simulink model "edrive"  (R2016b)
settings: Solver=ode1  StartTime=0.0  StopTime=1  FixedStep=ctrlConst.TsSim  MaxStep=1e-6  RelTol=1e-3  EnableMultiTasking=on
PreLoadFcn:
  | %rtwdemo_pmsmfoc_data
StartFcn:
  | %clear executionProfile
StopFcn:
  | %try
  | %  AddExecutionProfileToDataInspector();
  | %end
undefined symbols (not defined in the file or in its folder): canChannel, ctrlConst, ECM, EGM, hm11, hm13, hm5, hm7, Np, pmsm, sensors, sldrtexcb_modeswitch, SpdSetTest, theta0, TrqSetTest, Ts_10ms, Tsw
libraries: powerlib x26, canmsglib x23, simulink x14, canlib x12, powerlib_extras x9
(part 2 of 4)

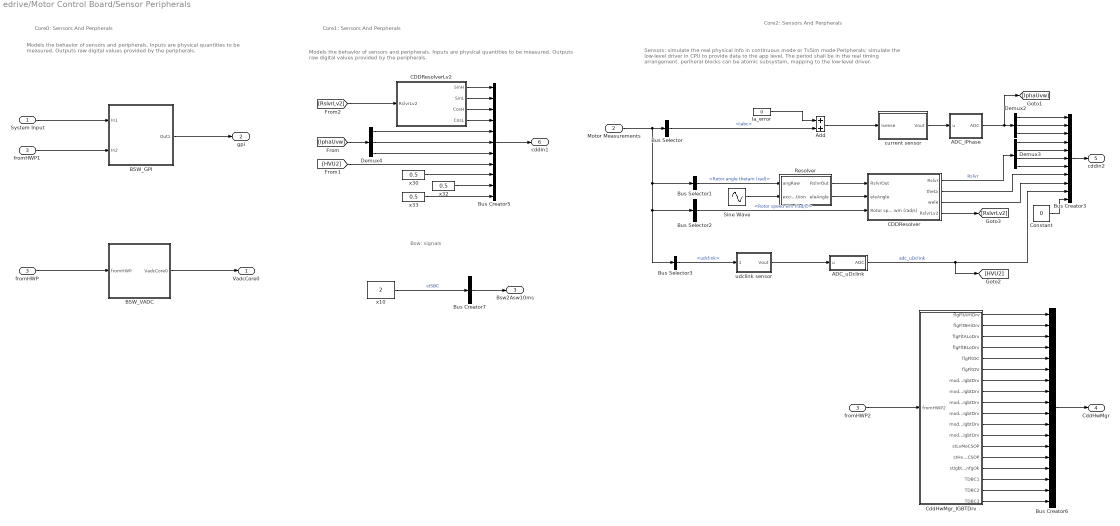
== system edrive/Motor Control Board/Sensor Peripherals ==
  note: Models the behavior of sensors and peripherals.
      | Inputs are physical quantities to be measured. Outputs raw digital values provided by the peripherals.
  note: Core0: Sensors And Perpherals
  note: Sensors: simulate the real physical info in continuous mode or TsSim mode
      | Peripherals: simulate the low-level driver in CPU to provide data to the app level. The period shall be in the real timing arrangement.
      | periheral blocks can be atomic subsystem, mapping to the low-level driver.
  note: Core2: Sensors And Perpherals
  note: Models the behavior of sensors and peripherals.
      | Inputs are physical quantities to be measured. Outputs raw digital values provided by the peripherals.
  note: Bsw: signals
  note: Core1: Sensors And Perpherals
  System Input : Inport
  Motor Measurements : Inport  Port=2
  fromHWP : Inport  Port=3
  ADC_iPhase : Subsystem
  ADC_uDclink : Subsystem
  Add : Sum
  BSW_GPI : Subsystem
  BSW_VADC : Subsystem
  Bus Creator3 : BusCreator  Inputs=11
  Bus Creator5 : BusCreator  Inputs=11
  Bus Creator6 : BusCreator  Inputs=18  OutDataTypeStr=Bus: CDDHwMgrST
  Bus Creator7 : BusCreator  Inputs=1
  Bus Selector : BusSelector  OutputSignals=electrical_measurements.Iabc
  Bus Selector1 : BusSelector  OutputSignals=mechanical_measurements.Rotor angle thetam (rad)
  Bus Selector2 : BusSelector  OutputSignals=mechanical_measurements.Rotor speed wm (rad/s)
  Bus Selector3 : BusSelector  OutputSignals=electrical_measurements.udclink
  CDDResolver : Subsystem
  CDDResolverLv2 : Subsystem
  CddHwMgr_IGBTDrv : Subsystem
  Constant : Constant  Value=0  OutDataTypeStr=uint16
  Demux2 : Demux  Outputs=3
  Demux3 : Demux
  Demux4 : Demux  Outputs=3
  Ia_error : Constant  Value=0
  Resolver : Subsystem
  Sine Wave : Sin  Amplitude=10  Frequency=10e3*2*pi  SampleTime=0
  current sensor : Subsystem
  fromHWP1 : InportShadow  Port=3
  fromHWP2 : InportShadow  Port=3
  udclink sensor : Subsystem
  x10 : Constant  Value=2  OutDataTypeStr=uint16
      settings: AttributesFormatString=DT: %<OutDataTypeStr>
  x30 : Constant  Value=0.5  OutDataTypeStr=single
      settings: AttributesFormatString=DT: %<OutDataTypeStr>
  x32 : Constant  Value=0.5  OutDataTypeStr=single
      settings: AttributesFormatString=DT: %<OutDataTypeStr>
  x33 : Constant  Value=0.5  OutDataTypeStr=single
      settings: AttributesFormatString=DT: %<OutDataTypeStr>
  VadcCore0 : Outport  OutDataTypeStr=Bus: VADCST
  gpi : Outport  Port=2  OutDataTypeStr=Bus: GPIST
  Bsw2Asw10ms : Outport  Port=3  OutDataTypeStr=Bus: Bsw2Asw10msST
  CddHwMgr : Outport  Port=4
  cddin2 : Outport  Port=5  OutDataTypeStr=Bus: CDDIN2ST
  cddin1 : Outport  Port=6  OutDataTypeStr=Bus: CDDIN1ST
  wires:
  Bus Creator6/1 -> CddHwMgr/1
  Bus Selector1/1 -> Resolver/1(angRaw)  "<Rotor angle thetam (rad)>"
  Sine Wave/1 -> Resolver/2(excitatiion)
  Motor Measurements/1 -> Bus Selector3/1, Bus Selector2/1, Bus Selector1/1, Bus Selector/1
  current sensor/1(Vout) -> ADC_iPhase/1(u)
  udclink sensor/1(Vout) -> ADC_uDclink/1(u)
  Bus Selector3/1 -> udclink sensor/1(uSense)  "<udclink>"
  Resolver/1(RslvrOut) -> CDDResolver/1(RslvrOut)
  Resolver/2(eleAngle) -> CDDResolver/2(eleAngle)
  Bus Selector2/1 -> CDDResolver/3(Rotor speed wm (rad/s))  "<Rotor speed wm (rad/s)>"
  Bus Selector/1 -> Add/2  "<Iabc>"
  ADC_uDclink/1(ADC) -> Bus Creator3/10, [HVU2]  "adc_uDclink"
  CDDResolver/1(Rslvr) -> Demux3/1  "Rslvr"
  Ia_error/1 -> Add/1
  Bus Creator5/1 -> cddin1/1
  [HVU2] -> Bus Creator5/8
  ADC_iPhase/1(ADC) -> [IphaUvw], Demux2/1
  [IphaUvw] -> Demux4/1
  Demux4/1 -> Bus Creator5/5
  Demux4/2 -> Bus Creator5/6
  Demux4/3 -> Bus Creator5/7
  CDDResolver/4(RslvrLv2) -> [RslvrLv2]
  CDDResolverLv2/1(SinH) -> Bus Creator5/1
  CDDResolverLv2/2(SinL) -> Bus Creator5/2
  CDDResolverLv2/3(CosH) -> Bus Creator5/3
  CDDResolverLv2/4(CosL) -> Bus Creator5/4
  [RslvrLv2] -> CDDResolverLv2/1(RslvrLv2)
  Bus Creator7/1 -> Bsw2Asw10ms/1
  x10/1 -> Bus Creator7/1  "stSBC"
  Add/1 -> current sensor/1(Isense)
  x30/1 -> Bus Creator5/9
  x32/1 -> Bus Creator5/10
  x33/1 -> Bus Creator5/11
  CddHwMgr_IGBTDrv/1(flgFltAHiDrv) -> Bus Creator6/1
  CddHwMgr_IGBTDrv/3(flgFltALoDrv) -> Bus Creator6/3
  CddHwMgr_IGBTDrv/4(flgFltBLoDrv) -> Bus Creator6/4
  CddHwMgr_IGBTDrv/5(flgFltOC) -> Bus Creator6/5
  CddHwMgr_IGBTDrv/6(flgFltOV) -> Bus Creator6/6
  CddHwMgr_IGBTDrv/13(stLvMoCSOP) -> Bus Creator6/13
  CddHwMgr_IGBTDrv/2(flgFltBHiDrv) -> Bus Creator6/2
  CddHwMgr_IGBTDrv/9(modLo3IgbtDrv) -> Bus Creator6/9
  CddHwMgr_IGBTDrv/12(modHi3IgbtDrv) -> Bus Creator6/12
  CddHwMgr_IGBTDrv/11(modHi2IgbtDrv) -> Bus Creator6/11
  CddHwMgr_IGBTDrv/7(modLo1IgbtDrv) -> Bus Creator6/7
  CddHwMgr_IGBTDrv/8(modLo2IgbtDrv) -> Bus Creator6/8
  CddHwMgr_IGBTDrv/10(modHi1IgbtDrv) -> Bus Creator6/10
  CddHwMgr_IGBTDrv/14(stHvMoCSOP) -> Bus Creator6/14
  BSW_VADC/1(VadcCore0) -> VadcCore0/1
  fromHWP/1 -> BSW_VADC/1(fromHWP)
  fromHWP2/1 -> CddHwMgr_IGBTDrv/1(fromHWP2)
  CddHwMgr_IGBTDrv/15(stIgbtDrvCnfgOk) -> Bus Creator6/15
  Bus Creator3/1 -> cddin2/1
  Demux2/1 -> Bus Creator3/1
  Demux2/2 -> Bus Creator3/2
  Demux2/3 -> Bus Creator3/3
  Demux3/1 -> Bus Creator3/4
  Demux3/2 -> Bus Creator3/5
  Demux3/3 -> Bus Creator3/6
  Demux3/4 -> Bus Creator3/7
  CDDResolver/2(theta) -> Bus Creator3/8
  CDDResolver/3(wele) -> Bus Creator3/9
  Constant/1 -> Bus Creator3/11
  CddHwMgr_IGBTDrv/16(TDBC1) -> Bus Creator6/16
  CddHwMgr_IGBTDrv/17(TDBC2) -> Bus Creator6/17
  CddHwMgr_IGBTDrv/18(TDBC3) -> Bus Creator6/18
  System Input/1 -> BSW_GPI/1(In1)
  fromHWP1/1 -> BSW_GPI/2(In2)
  BSW_GPI/1(Out1) -> gpi/1

== system edrive/Power Inverter and Motor/Inverter ==
  note: Change UVW to Motor here
  note: Construct electrical waveforms for the three motor phases.
  note: Inverter
  gate1 : Inport
  Bus Creator : BusCreator  Inputs=3
  Current Measurement : powerlib/Measurements/Current Measurement  Tag=PoWeRsYsTeMmEaSuReMeNt  PhasorSimulation=off  OutputType=Magnitude  PSBequivalent=0
  DC Voltage Source1 : powerlib/Electrical Sources/DC Voltage Source  Amplitude=pmsm.Udc  Measurements=None
  IGBT  B6 : powerlib/Power Electronics/Universal Bridge  Arms=3  SnubberResistance=1e6  SnubberCapacitance=1e-9  Device=IGBT / Diodes  Ron=1.1e-3  Lon=0  ForwardVoltages="[0.7  0.7]"  ForwardVoltage=0  GTOparameters=[ 10e-6 , 20e-6 ]  IGBTparameters=[0.1e-6 , 0.1e-6 ]  Measurements=None  Measurements_2=None  converterType=Rectifier
  Measure : Subsystem
  RC1 : powerlib/Elements/Series RLC Branch  LConnTagsString=__new0  RConnTagsString=__new0  BranchType=RC  Resistance=0.001  Inductance=7e-9  SetiL0=off  InitialCurrent=0  Capacitance=500e-6  Setx0=on  InitialVoltage=pmsm.Udc  Measurements=None
  RC2 : powerlib/Elements/Series RLC Branch  LConnTagsString=__new0  RConnTagsString=__new0  BranchType=RL  Resistance=(45+2)*1e-3  Inductance=2.5e-6  SetiL0=off  InitialCurrent=0  Capacitance=500e-6  Setx0=off  InitialVoltage=0  Measurements=None
  Rshort : powerlib/Elements/Series RLC Branch  LConnTagsString=__new0  RConnTagsString=__new0  BranchType=R  Resistance=1e-5  Inductance=7e-9  SetiL0=off  InitialCurrent=0  Capacitance=500e-6  Setx0=on  InitialVoltage=330  Measurements=None
  A : PMIOPort  Port=1  Side=Right
  B : PMIOPort  Port=2  Side=Right
  C : PMIOPort  Port=3  Side=Right
  "EleMeasurement " : Outport
  wires:
  Current Measurement/1 -> Measure/1(Idc)
  Measure/2(I_abc) -> Bus Creator/2  "Iabc"
  Measure/3(Vdc) -> Bus Creator/3  "udclink"
  gate1/1 -> IGBT  B6/1
  Bus Creator/1 -> "EleMeasurement "/1
  Measure/1(Pdclnk) -> Bus Creator/1  "Pdclink"
  connections:
  DC Voltage Source1/LConn1 -- IGBT  B6/RConn2 -- Measure/LConn4 -- RC1/RConn1
  RC2/LConn1 -- RC1/LConn1 -- Measure/LConn5 -- Current Measurement/LConn1 -- Rshort/LConn1
  DC Voltage Source1/RConn1 -- RC2/RConn1 -- Rshort/RConn1
  A/RConn1 -- Measure/RConn1
  IGBT  B6/RConn1 -- Current Measurement/RConn1
  Measure/RConn2 -- B/RConn1
  Measure/RConn3 -- C/RConn1
  IGBT  B6/LConn2 -- Measure/LConn2
  IGBT  B6/LConn1 -- Measure/LConn1
  IGBT  B6/LConn3 -- Measure/LConn3

== system edrive/Power Inverter and Motor/Motor_feishi150 ==
  note: Motor
  note: Models the PMSM and outputs physical quantities used by the controller and visualizations.
      | The rotor position angle returned by the SimPowerSystems model must be offset to align with the reference angle that the controller expects.
      | Signal conversion blocks are used to enable renaming signals measured from the motor model.
  MotorMode : Inport
  Speed or Torque : Inport  Port=2
  Gain12 : Gain  Gain=2*pi/60
  PMSM : Subsystem
  A : PMIOPort  Port=1  Side=Left
  B : PMIOPort  Port=2  Side=Left
  C : PMIOPort  Port=3  Side=Left
  MotorMeasure : Outport
  wires:
  Speed or Torque/1 -> Gain12/1
  PMSM/1(m) -> MotorMeasure/1
  Gain12/1 -> PMSM/1(In)
  MotorMode/1 -> PMSM/2(MotorMode)
  connections:
  PMSM/LConn3 -- C/RConn1
  PMSM/LConn2 -- B/RConn1
  PMSM/LConn1 -- A/RConn1

== system edrive/System Analysis/Measure ==
  motor : Inport
  Bus Selector1 : BusSelector  OutputSignals=mechanical_measurements.Stator current is_q (A),mechanical_measurements.Stator current is_d (A),mechanical_measurements.Stator voltage Vs_q (V),mechanical_measurements.Stator voltage Vs_d (V),mechanical_measurements.Rotor speed wm (rad/s),mechanical_measurements.Electromagnetic torque Te (N*m),electrical_measurements.Pdclink
  Eff Cal : MATLAB Function  TreatAsAtomicUnit=on
  Gain : Gain  Gain=1/sqrt(2)
  Gain1 : Gain  Gain=1/sqrt(2)
  Loss : Scope  NumInputPorts=2
  Mux2 : Mux  Inputs=2
  Saturation : Saturate  UpperLimit=1  LowerLimit=0
  Subsystem : Subsystem
  Subsystem1 : Subsystem
  Subsystem3 : Subsystem
  Subsystem4 : Subsystem
  Transfer Fcn1 : TransferFcn  Numerator=[1/sqrt(2)]  Denominator=[0.001 1]
  Transfer Fcn2 : TransferFcn  Denominator=[0.01 1]
  Transfer Fcn3 : TransferFcn  Numerator=[1/sqrt(2)]  Denominator=[0.001 1]
  Torque : Outport
  speed : Outport  Port=2
  Current : Outport  Port=3
  Voltage : Outport  Port=4
  Power : Outport  Port=5
  effEDrive : Outport  Port=6
  wires:
  motor/1 -> Bus Selector1/1
  Bus Selector1/2 -> Gain1/1  "<Stator current is_d (A)>"
  Bus Selector1/1 -> Gain/1  "<Stator current is_q (A)>"
  Bus Selector1/4 -> Transfer Fcn1/1  "<Stator voltage Vs_d (V)>"
  Bus Selector1/3 -> Transfer Fcn3/1  "<Stator voltage Vs_q (V)>"
  Subsystem/1(Cur.) -> Current/1
  Subsystem1/1(Vol.) -> Voltage/1
  Transfer Fcn3/1 -> Subsystem3/2(vq), Subsystem1/1(vq)
  Transfer Fcn1/1 -> Subsystem1/2(vd), Subsystem3/1(vd)
  Bus Selector1/5 -> Subsystem4/1(In1)  "<Rotor speed wm (rad/s)>"
  Bus Selector1/6 -> Subsystem4/2(In2)  "<Electromagnetic torque Te (N*m)>"
  Subsystem4/1(Torque) -> Torque/1
  Subsystem4/2(speed) -> speed/1
  Gain/1 -> Subsystem3/4(iq), Subsystem/1(iq)
  Gain1/1 -> Subsystem/2(id), Subsystem3/3(id)
  Mux2/1 -> Power/1
  Subsystem4/3(M_Power) -> Eff Cal/1(m_power), Mux2/1
  Saturation/1 -> Loss/1, effEDrive/1
  Eff Cal/1(eff) -> Saturation/1
  Bus Selector1/7 -> Transfer Fcn2/1  "<Pdclink>"
  Transfer Fcn2/1 -> Loss/2, Mux2/2, Eff Cal/2(e_power)

== system edrive/System Analysis/System test ==
  torque_in : Inport
  Abs : Abs
  Data Type Conversion2 : DataTypeConversion  OutDataTypeStr=double
  Demux : Demux  Outputs=2
  Rate Transition1 : RateTransition  OutPortSampleTime=0.001
  Rate Transition2 : RateTransition  OutPortSampleTime=1e-2
  Rate Transition4 : RateTransition  OutPortSampleTime=1e-2
  Subtract : Sum  Inputs=-+
  To TrqErrRms : ToWorkspace  VariableName=TrqErrRms  SaveFormat=Timeseries  SampleTime=0.001
      settings: MaxDataPoints=50
  test : MATLAB Function  TreatAsAtomicUnit=on  SystemSampleTime=1e-2
  Out : Outport
  wires:
  test/1(out) -> Out/1
  Demux/2 -> Data Type Conversion2/1, Rate Transition4/1
  torque_in/1 -> Demux/1
  Subtract/1 -> Abs/1
  Abs/1 -> Rate Transition1/1
  Rate Transition4/1 -> test/2(torque_act)
  Data Type Conversion2/1 -> Subtract/2
  Demux/1 -> Rate Transition2/1, Subtract/1
  Rate Transition1/1 -> To TrqErrRms/1
  Rate Transition2/1 -> test/1(torqueSet)

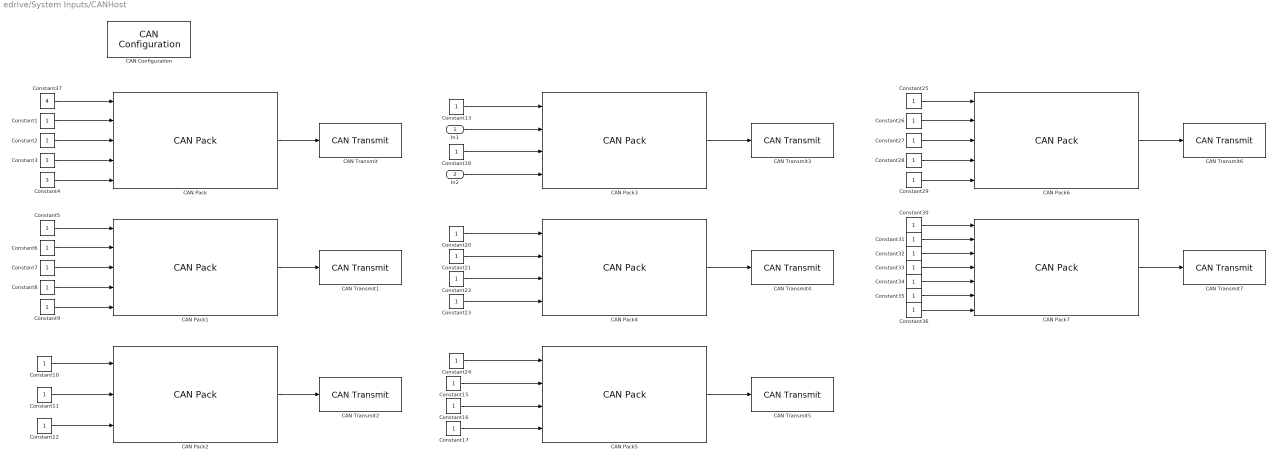
== system edrive/System Inputs/CANHost ==
  In1 : Inport
  In2 : Inport  Port=2
  CAN Configuration : canlib/CAN Configuration  BlockHandle=9440.0004  DeviceMenu=Kvaser Virtual 1 (Channel 2)  Device=Kvaser Virtual 1 (Channel 2)  ObjConstructor=canChannel('Kvaser', 'Virtual 1', 2)  BusSpeed=500000  EnableBitParameters=off  SJW=1  TSEG1=4  TSEG2=3  NSamples=1  AckMode=Normal
  CAN Pack : canmsglib/CAN Pack  CANdbFile=C:\MatlabWS\motorcontrol\controller\CAN_COM.dbc  MsgList=MSG_01  MsgName=MSG_01  MsgIDType=Standard (11-bit identifier)  MsgIdentifier=768  MsgLength=8  SignalInfo=MSG01_IdcMax$0$11$1$2$1$0$1$-1023$-1023$1024$#MSG01_IdcMin$11$11$1$2$1$0$1$-1023$-1023$1024$#MSG01_UdcMax$22$10$1$2$1$0$1$0$0$1023$#MSG01_UdcMin$32$10$1$2$1$0$1$0$0$1023$#MSG01_stHvbMaiRly$42$3$1$2$1$0$1$0$0$7$#  NSignals=5  StartBits=str2num('[int32(0);int32(11);int32(22);int32(32);int32(42)]')  SignalSizes=str2num('[int32(11);int32(11);int32(10);int32(10);int32(3)]')  ByteOrders=str2num('[int32(1);int32(1);int32(1);int32(1);int32(1)]')  DataTypes=str2num('[int32(2);int32(2);int32(2);int32(2);int32(2)]')  MultiplexTypes=str2num('[int32(1);int32(1);int32(1);int32(1);int32(1)]')  MultiplexValues=str2num('[double(0);double(0);double(0);double(0);double(0)]')  Factors=str2num('[double(1);double(1);double(1);double(1);double(1)]')  Offsets=str2num('[double(-1023);double(-1023);double(0);double(0);double(0)]')  Minimums=str2num('[double(-1023);double(-1023);double(0);double(0);double(0)]')  Maximums=str2num('[double(1024);double(1024);double(1023);double(1023);double(7)]')  Remote=off
      settings: DataFormat=CANdb specified signals
  CAN Pack1 : canmsglib/CAN Pack  CANdbFile=C:\MatlabWS\motorcontrol\controller\CAN_COM.dbc  MsgList=MSG_02  MsgName=MSG_02  MsgIDType=Standard (11-bit identifier)  MsgIdentifier=784  MsgLength=8  SignalInfo=MSG02_KpHigh$0$9$1$2$1$0$3.125000e-02$0$0$10$#MSG02_KpLow$9$9$1$2$1$0$3.125000e-02$0$0$10$#MSG02_NDeltaBound$18$16$1$2$1$0$5.000000e-01$-1.638350e+04$-1.638350e+04$16384$#MSG02_TrqPAmax$45$11$1$2$1$0$1$-1023$-1023$1024$#MSG02_TrqPAmin$34$11$1$2$1$0$1$-1023$-1023$1024$#  NSignals=5  StartBits=str2num('[int32(0);int32(9);int32(18);int32(45);int32(34)]')  SignalSizes=str2num('[int32(9);int32(9);int32(16);int32(11);int32(11)]')  ByteOrders=str2num('[int32(1);int32(1);int32(1);int32(1);int32(1)]')  DataTypes=str2num('[int32(2);int32(2);int32(2);int32(2);int32(2)]')  MultiplexTypes=str2num('[int32(1);int32(1);int32(1);int32(1);int32(1)]')  MultiplexValues=str2num('[double(0);double(0);double(0);double(0);double(0)]')  Factors=str2num('[double(3.125000e-02);double(3.125000e-02);double(5.000000e-01);double(1);double(1)]')  Offsets=str2num('[double(0);double(0);double(-1.638350e+04);double(-1023);double(-1023)]')  Minimums=str2num('[double(0);double(0);double(-1.638350e+04);double(-1023);double(-1023)]')  Maximums=str2num('[double(10);double(10);double(16384);double(1024);double(1024)]')  Remote=off
      settings: DataFormat=CANdb specified signals
  CAN Pack2 : canmsglib/CAN Pack  CANdbFile=C:\MatlabWS\motorcontrol\controller\CAN_COM.dbc  MsgList=MSG_03  MsgName=MSG_03  MsgIDType=Standard (11-bit identifier)  MsgIdentifier=800  MsgLength=8  SignalInfo=MSG03_TrqMax$0$11$1$2$1$0$1$-1023$-1023$1024$#MSG03_TrqMin$11$11$1$2$1$0$1$-1023$-1023$1024$#MSG03_cTrqSlopeMax$24$15$1$2$1$0$32$0$0$1048544$#  NSignals=3  StartBits=str2num('[int32(0);int32(11);int32(24)]')  SignalSizes=str2num('[int32(11);int32(11);int32(15)]')  ByteOrders=str2num('[int32(1);int32(1);int32(1)]')  DataTypes=str2num('[int32(2);int32(2);int32(2)]')  MultiplexTypes=str2num('[int32(1);int32(1);int32(1)]')  MultiplexValues=str2num('[double(0);double(0);double(0)]')  Factors=str2num('[double(1);double(1);double(32)]')  Offsets=str2num('[double(-1023);double(-1023);double(0)]')  Minimums=str2num('[double(-1023);double(-1023);double(0)]')  Maximums=str2num('[double(1024);double(1024);double(1048544)]')  Remote=off
      settings: DataFormat=CANdb specified signals
  CAN Pack3 : canmsglib/CAN Pack  CANdbFile=C:\MatlabWS\motorcontrol\controller\CAN_COM.dbc  MsgList=MSG_04  MsgName=MSG_04  MsgIDType=Standard (11-bit identifier)  MsgIdentifier=256  MsgLength=8  SignalInfo=MSG04_NSetP$0$16$1$2$1$0$1$-32767$-32767$32768$#MSG04_TrqSetP$20$11$1$2$1$0$1$-1023$-1023$1024$#MSG04_UdcSetP$32$10$1$2$1$0$1$0$0$1023$#MSG04_stModeReq$16$4$1$2$1$0$1$0$0$15$#  NSignals=4  StartBits=str2num('[int32(0);int32(20);int32(32);int32(16)]')  SignalSizes=str2num('[int32(16);int32(11);int32(10);int32(4)]')  ByteOrders=str2num('[int32(1);int32(1);int32(1);int32(1)]')  DataTypes=str2num('[int32(2);int32(2);int32(2);int32(2)]')  MultiplexTypes=str2num('[int32(1);int32(1);int32(1);int32(1)]')  MultiplexValues=str2num('[double(0);double(0);double(0);double(0)]')  Factors=str2num('[double(1);double(1);double(1);double(1)]')  Offsets=str2num('[double(-32767);double(-1023);double(0);double(0)]')  Minimums=str2num('[double(-32767);double(-1023);double(0);double(0)]')  Maximums=str2num('[double(32768);double(1024);double(1023);double(15)]')  Remote=off
      settings: DataFormat=CANdb specified signals
  CAN Pack4 : canmsglib/CAN Pack  CANdbFile=C:\MatlabWS\motorcontrol\controller\CAN_COM.dbc  MsgList=EM_05  MsgName=EM_05  MsgIDType=Standard (11-bit identifier)  MsgIdentifier=576  MsgLength=8  SignalInfo=EM05_FailCode1$0$16$1$2$1$0$1$0$0$65535$#EM05_FailCode2$16$16$1$2$1$0$1$0$0$65535$#EM05_FailCode3$32$16$1$2$1$0$1$0$0$65535$#EM05_FailCode4$48$16$1$2$1$0$1$0$0$65535$#  NSignals=4  StartBits=str2num('[int32(0);int32(16);int32(32);int32(48)]')  SignalSizes=str2num('[int32(16);int32(16);int32(16);int32(16)]')  ByteOrders=str2num('[int32(1);int32(1);int32(1);int32(1)]')  DataTypes=str2num('[int32(2);int32(2);int32(2);int32(2)]')  MultiplexTypes=str2num('[int32(1);int32(1);int32(1);int32(1)]')  MultiplexValues=str2num('[double(0);double(0);double(0);double(0)]')  Factors=str2num('[double(1);double(1);double(1);double(1)]')  Offsets=str2num('[double(0);double(0);double(0);double(0)]')  Minimums=str2num('[double(0);double(0);double(0);double(0)]')  Maximums=str2num('[double(65535);double(65535);double(65535);double(65535)]')  Remote=off
      settings: DataFormat=CANdb specified signals
  CAN Pack5 : canmsglib/CAN Pack  CANdbFile=C:\MatlabWS\motorcontrol\controller\CAN_COM.dbc  MsgList=MSG_06  MsgName=MSG_06  MsgIDType=Standard (11-bit identifier)  MsgIdentifier=288  MsgLength=8  SignalInfo=MSG06_TrqDmpLim$12$10$1$2$1$0$1$0$0$1023$#MSG06_TrqDmpMax$2$10$1$2$1$0$1$0$0$1023$#MSG06_kDmp$24$15$1$2$1$0$3.125000e-02$0$0$8$#MSG06_stDstCReq$0$2$1$2$1$0$1$0$0$3$#  NSignals=4  StartBits=str2num('[int32(12);int32(2);int32(24);int32(0)]')  SignalSizes=str2num('[int32(10);int32(10);int32(15);int32(2)]')  ByteOrders=str2num('[int32(1);int32(1);int32(1);int32(1)]')  DataTypes=str2num('[int32(2);int32(2);int32(2);int32(2)]')  MultiplexTypes=str2num('[int32(1);int32(1);int32(1);int32(1)]')  MultiplexValues=str2num('[double(0);double(0);double(0);double(0)]')  Factors=str2num('[double(1);double(1);double(3.125000e-02);double(1)]')  Offsets=str2num('[double(0);double(0);double(0);double(0)]')  Minimums=str2num('[double(0);double(0);double(0);double(0)]')  Maximums=str2num('[double(1023);double(1023);double(8);double(3)]')  Remote=off
      settings: DataFormat=CANdb specified signals
  CAN Pack6 : canmsglib/CAN Pack  CANdbFile=C:\MatlabWS\motorcontrol\controller\CAN_COM.dbc  MsgList=MSG_01  MsgName=MSG_01  MsgIDType=Standard (11-bit identifier)  MsgIdentifier=768  MsgLength=8  SignalInfo=MSG01_IdcMax$0$11$1$2$1$0$1$-1023$-1023$1024$#MSG01_IdcMin$11$11$1$2$1$0$1$-1023$-1023$1024$#MSG01_UdcMax$22$10$1$2$1$0$1$0$0$1023$#MSG01_UdcMin$32$10$1$2$1$0$1$0$0$1023$#MSG01_stHvbMaiRly$42$3$1$2$1$0$1$0$0$7$#  NSignals=5  StartBits=str2num('[int32(0);int32(11);int32(22);int32(32);int32(42)]')  SignalSizes=str2num('[int32(11);int32(11);int32(10);int32(10);int32(3)]')  ByteOrders=str2num('[int32(1);int32(1);int32(1);int32(1);int32(1)]')  DataTypes=str2num('[int32(2);int32(2);int32(2);int32(2);int32(2)]')  MultiplexTypes=str2num('[int32(1);int32(1);int32(1);int32(1);int32(1)]')  MultiplexValues=str2num('[double(0);double(0);double(0);double(0);double(0)]')  Factors=str2num('[double(1);double(1);double(1);double(1);double(1)]')  Offsets=str2num('[double(-1023);double(-1023);double(0);double(0);double(0)]')  Minimums=str2num('[double(-1023);double(-1023);double(0);double(0);double(0)]')  Maximums=str2num('[double(1024);double(1024);double(1023);double(1023);double(7)]')  Remote=off
      settings: DataFormat=CANdb specified signals
  CAN Pack7 : canmsglib/CAN Pack  CANdbFile=C:\MatlabWS\motorcontrol\controller\CAN_COM.dbc  MsgList=MSG_08  MsgName=MSG_08  MsgIDType=Extended (29-bit identifier)  MsgIdentifier=320  MsgLength=7  SignalInfo=MSG08_Alpha_Voltage_Cmd$8$8$1$2$1$0$1$0$0$255$#MSG08_Beta_Voltage_Cmd$16$8$1$2$1$0$1$0$0$255$#MSG08_D_Current_Cmd$48$8$1$2$1$0$1$0$0$255$#MSG08_D_Voltage_Cmd$24$8$1$2$1$0$1$0$0$255$#MSG08_Q_Current_Cmd$40$8$1$2$1$0$1$0$0$255$#MSG08_Q_Volatge_Cmd$32$8$1$2$1$0$1$0$0$255$#MSG08_control_mode$0$3$1$2$1$0$1$0$0$7$#  NSignals=7  StartBits=str2num('[int32(8);int32(16);int32(48);int32(24);int32(40);int32(32);int32(0)]')  SignalSizes=str2num('[int32(8);int32(8);int32(8);int32(8);int32(8);int32(8);int32(3)]')  ByteOrders=str2num('[int32(1);int32(1);int32(1);int32(1);int32(1);int32(1);int32(1)]')  DataTypes=str2num('[int32(2);int32(2);int32(2);int32(2);int32(2);int32(2);int32(2)]')  MultiplexTypes=str2num('[int32(1);int32(1);int32(1);int32(1);int32(1);int32(1);int32(1)]')  MultiplexValues=str2num('[double(0);double(0);double(0);double(0);double(0);double(0);double(0)]')  Factors=str2num('[double(1);double(1);double(1);double(1);double(1);double(1);double(1)]')  Offsets=str2num('[double(0);double(0);double(0);double(0);double(0);double(0);double(0)]')  Minimums=str2num('[double(0);double(0);double(0);double(0);double(0);double(0);double(0)]')  Maximums=str2num('[double(255);double(255);double(255);double(255);double(255);double(255);double(7)]')  Remote=off
      settings: DataFormat=CANdb specified signals
  CAN Transmit : canlib/CAN Transmit  BlockHandle=9449.0004  DeviceMenu=Kvaser Virtual 1 (Channel 2)  Device=Kvaser Virtual 1 (Channel 2)  ObjConstructor=canChannel('Kvaser', 'Virtual 1', 2)  EnablePeriodicTransmit=on  MessagePeriod=0.01
  CAN Transmit1 : canlib/CAN Transmit  BlockHandle=9450.0004  DeviceMenu=Kvaser Virtual 1 (Channel 2)  Device=Kvaser Virtual 1 (Channel 2)  ObjConstructor=canChannel('Kvaser', 'Virtual 1', 2)  EnablePeriodicTransmit=on  MessagePeriod=0.01
  CAN Transmit2 : canlib/CAN Transmit  BlockHandle=9451.0004  DeviceMenu=Kvaser Virtual 1 (Channel 2)  Device=Kvaser Virtual 1 (Channel 2)  ObjConstructor=canChannel('Kvaser', 'Virtual 1', 2)  EnablePeriodicTransmit=on  MessagePeriod=0.01
  CAN Transmit3 : canlib/CAN Transmit  BlockHandle=9452.0004  DeviceMenu=Kvaser Virtual 1 (Channel 2)  Device=Kvaser Virtual 1 (Channel 2)  ObjConstructor=canChannel('Kvaser', 'Virtual 1', 2)  EnablePeriodicTransmit=on  MessagePeriod=0.01
  CAN Transmit4 : canlib/CAN Transmit  BlockHandle=9453.0004  DeviceMenu=Kvaser Virtual 1 (Channel 2)  Device=Kvaser Virtual 1 (Channel 2)  ObjConstructor=canChannel('Kvaser', 'Virtual 1', 2)  EnablePeriodicTransmit=on  MessagePeriod=0.01
  CAN Transmit5 : canlib/CAN Transmit  BlockHandle=9454.0004  DeviceMenu=Kvaser Virtual 1 (Channel 2)  Device=Kvaser Virtual 1 (Channel 2)  ObjConstructor=canChannel('Kvaser', 'Virtual 1', 2)  EnablePeriodicTransmit=on  MessagePeriod=0.01
  CAN Transmit6 : canlib/CAN Transmit  BlockHandle=9455.0004  DeviceMenu=Kvaser Virtual 1 (Channel 2)  Device=Kvaser Virtual 1 (Channel 2)  ObjConstructor=canChannel('Kvaser', 'Virtual 1', 2)  EnablePeriodicTransmit=on  MessagePeriod=0.01
  CAN Transmit7 : canlib/CAN Transmit  BlockHandle=9456.0004  DeviceMenu=Kvaser Virtual 1 (Channel 2)  Device=Kvaser Virtual 1 (Channel 2)  ObjConstructor=canChannel('Kvaser', 'Virtual 1', 2)  EnablePeriodicTransmit=on  MessagePeriod=0.01
  Constant{1..3,5..13,15..18,20..36} (33 alike) : Constant
  Constant37 : Constant  Value=4
  Constant4 : Constant  Value=3
  wires:
  CAN Pack/1 -> CAN Transmit/1
  CAN Pack1/1 -> CAN Transmit1/1
  CAN Pack2/1 -> CAN Transmit2/1
  CAN Pack3/1 -> CAN Transmit3/1
  CAN Pack4/1 -> CAN Transmit4/1
  CAN Pack5/1 -> CAN Transmit5/1
  CAN Pack6/1 -> CAN Transmit6/1
  CAN Pack7/1 -> CAN Transmit7/1
  Constant37/1 -> CAN Pack/1
  Constant1/1 -> CAN Pack/2
  Constant2/1 -> CAN Pack/3
  Constant3/1 -> CAN Pack/4
  Constant4/1 -> CAN Pack/5
  Constant7/1 -> CAN Pack1/3
  Constant8/1 -> CAN Pack1/4
  Constant6/1 -> CAN Pack1/2
  Constant9/1 -> CAN Pack1/5
  Constant5/1 -> CAN Pack1/1
  Constant11/1 -> CAN Pack2/2
  Constant10/1 -> CAN Pack2/1
  Constant12/1 -> CAN Pack2/3
  Constant13/1 -> CAN Pack3/1
  In1/1 -> CAN Pack3/2
  Constant18/1 -> CAN Pack3/3
  In2/1 -> CAN Pack3/4
  Constant21/1 -> CAN Pack4/2
  Constant22/1 -> CAN Pack4/3
  Constant23/1 -> CAN Pack4/4
  Constant20/1 -> CAN Pack4/1
  Constant17/1 -> CAN Pack5/4
  Constant16/1 -> CAN Pack5/3
  Constant24/1 -> CAN Pack5/1
  Constant15/1 -> CAN Pack5/2
  Constant28/1 -> CAN Pack6/4
  Constant26/1 -> CAN Pack6/2
  Constant27/1 -> CAN Pack6/3
  Constant29/1 -> CAN Pack6/5
  Constant25/1 -> CAN Pack6/1
  Constant31/1 -> CAN Pack7/2
  Constant30/1 -> CAN Pack7/1
  Constant32/1 -> CAN Pack7/3
  Constant33/1 -> CAN Pack7/4
  Constant34/1 -> CAN Pack7/5
  Constant35/1 -> CAN Pack7/6
  Constant36/1 -> CAN Pack7/7

== system edrive/Motor Control Board/ComCanRxdGen/Subsystem1 ==
  In1 : Inport
  Terminator : Terminator
  Out1 : Outport
  wires:
  In1/1 -> Terminator/1
  [TrqInCan] -> Out1/1

== system edrive/Motor Control Board/ComCanRxdGen/Subsystem2 ==
  In1 : Inport
  Terminator : Terminator
  Out1 : Outport
  wires:
  [ModeInCan] -> Out1/1
  In1/1 -> Terminator/1

== system edrive/Motor Control Board/ComCanRxdGen/Subsystem3 ==
  In1 : Inport
  Terminator : Terminator
  Out1 : Outport
  wires:
  In1/1 -> Terminator/1
  [SpdInCan] -> Out1/1

== system edrive/Motor Control Board/GTM/SVPWMtoDuty ==
  note: Hoang Le-Huy
      | Universite Laval
      | Quebec
  note: Pierre Giroux, Gilbert Sybille
      | Power System Laboratory, IREQ
      | Hydro-Quebec
  note: Space Vector Pulse Width Modulation (SV PWM)
  tSwitch : Inport
  Demux2 : Demux  Outputs=12
  Generate pulse pattern : Subsystem
      mask init:
      | %Switching pattern:
      | pat1=[0 1 1 1 1 1 0;0 0 1 1 1 0 0;0 0 0 1 0 0 0];
      | pat1(:,:,2)=[0 0 1 1 1 0 0;0 1 1 1 1 1 0;0 0 0 1 0 0 0];
      | pat1(:,:,3)=[0 0 0 1 0 0 0;0 1 1 1 1 1 0;0 0 1 1 1 0 0];
      | pat1(:,:,4)=[0 0 0 1 0 0 0;0 0 1 1 1 0 0;0 1 1 1 1 1 0];
      | pat1(:,:,5)=[0 0 1 1 1 0 0;0 0 0 1 0 0 0;0 1 1 1 1 1 0];
      | pat1(:,:,6)=[0 1 1 1 1 1 0;0 0 0 1 0 0 0;0 0 1 1 1 0 0];
  Generate pulse pattern1 : Subsystem
      mask init: same as edrive/Motor Control Board/GTM/SVPWMtoDuty/Generate pulse pattern
  Generate pulse pattern2 : Subsystem
      mask init: same as edrive/Motor Control Board/GTM/SVPWMtoDuty/Generate pulse pattern
  Generate pulse pattern3 : Subsystem
      mask init: same as edrive/Motor Control Board/GTM/SVPWMtoDuty/Generate pulse pattern
  Generate pulse pattern4 : Subsystem
      mask init: same as edrive/Motor Control Board/GTM/SVPWMtoDuty/Generate pulse pattern
  Generate pulse pattern5 : Subsystem
      mask init: same as edrive/Motor Control Board/GTM/SVPWMtoDuty/Generate pulse pattern
  INFO : Subsystem
      mask Display: disp('?')
  Mux : Mux  Inputs=6
  Pulses : Outport
  wires:
  Generate pulse pattern5/1(TuLo) -> Mux/6
  Generate pulse pattern4/1(TuLo) -> Mux/4
  Generate pulse pattern1/1(TuHi) -> Mux/3
  Generate pulse pattern/1(TuHi) -> Mux/1
  Demux2/12 -> Generate pulse pattern5/2(TuLo_On)
  Demux2/11 -> Generate pulse pattern5/1(TuLo_Off)
  Demux2/10 -> Generate pulse pattern4/2(TuLo_On)
  Demux2/9 -> Generate pulse pattern4/1(TuLo_Off)
  Demux2/8 -> Generate pulse pattern3/2(TuLo_On)
  Demux2/7 -> Generate pulse pattern3/1(TuLo_Off)
  Demux2/6 -> Generate pulse pattern2/2(TuHi_Off)
  Demux2/5 -> Generate pulse pattern2/1(TuHi_On)
  Demux2/4 -> Generate pulse pattern1/2(TuHi_Off)
  Demux2/3 -> Generate pulse pattern1/1(TuHi_On)
  Demux2/2 -> Generate pulse pattern/2(TuHi_Off)
  Demux2/1 -> Generate pulse pattern/1(TuHi_On)
  tSwitch/1 -> Demux2/1
  Mux/1 -> Pulses/1
  Generate pulse pattern3/1(TuLo) -> Mux/2
  Generate pulse pattern2/1(TuHi) -> Mux/5

== system edrive/Motor Control Board/Sensor Peripherals/ADC_iPhase ==
  u : Inport
  ADC Volts To Driver Units : Constant  Value=sensors.ADC.VoltsToDriverUnits
  Driver Noise : Subsystem
      mask init:
      | if evalin('base','sensors.ADC.NoiseEnable')
      |     enable = 'Enabled';
      | else
      |     enable = 'Disabled';
      | end
      mask Display: fprintf(['ADC Driver Noise\n(' enable ')'])
  Gain : Gain  Gain=16  ParamDataTypeStr=uint16  OutDataTypeStr=uint16
  Product Volts To Driver Units : Product  RndMeth=Zero
  Saturation : Saturate  UpperLimit=sensors.ADC.MaxDriverUnits  LowerLimit=0  OutDataTypeStr=uint16
      settings: AttributesFormatString=----------------------------\nUpper Limit: %<UpperLimit>\nLower Limit: %<LowerLimit>
  ADC : Outport  OutDataTypeStr=uint16
  wires:
  u/1 -> Product Volts To Driver Units/1
  ADC Volts To Driver Units/1 -> Product Volts To Driver Units/2
  Product Volts To Driver Units/1 -> Saturation/1
  Saturation/1 -> Driver Noise/1(In)
  Driver Noise/1(Out) -> Gain/1
  Gain/1 -> ADC/1  "adc_iPhase"

== system edrive/Motor Control Board/Sensor Peripherals/ADC_uDclink ==
  u : Inport
  ADC Volts To Driver Units : Constant  Value=sensors.ADC.VoltsToDriverUnits
  Driver Noise : Subsystem
      mask init:
      | if evalin('base','sensors.ADC.NoiseEnable')
      |     enable = 'Enabled';
      | else
      |     enable = 'Disabled';
      | end
      mask Display: fprintf(['ADC Driver Noise\n(' enable ')'])
  Gain : Gain  Gain=16  ParamDataTypeStr=uint16  OutDataTypeStr=uint16
  Product Volts To Driver Units : Product  RndMeth=Zero
  Saturation : Saturate  UpperLimit=sensors.ADC.MaxDriverUnits  LowerLimit=0  OutDataTypeStr=uint16
      settings: AttributesFormatString=----------------------------\nUpper Limit: %<UpperLimit>\nLower Limit: %<LowerLimit>
  ADC : Outport  OutDataTypeStr=uint16
  wires:
  Gain/1 -> ADC/1  "adc_uDclink"
  Driver Noise/1(Out) -> Gain/1
  Saturation/1 -> Driver Noise/1(In)
  Product Volts To Driver Units/1 -> Saturation/1
  ADC Volts To Driver Units/1 -> Product Volts To Driver Units/2
  u/1 -> Product Volts To Driver Units/1

== system edrive/Motor Control Board/Sensor Peripherals/BSW_GPI ==
  In1 : Inport
  In2 : Inport  Port=2
  Bus Creator1 : BusCreator  Inputs=5
  Bus Selector4 : BusSelector  OutputSignals=kl15
  Bus Selector5 : BusSelector  OutputSignals=RDY_H,RDY_L
  Bus Selector6 : BusSelector  OutputSignals=kl15,RDY_H,RDY_L,stL2AscEn,wake  OutputAsBus=on
  x2 : Constant  Value=0  OutDataTypeStr=boolean
      settings: AttributesFormatString=DT: %<OutDataTypeStr>
  x6 : Constant  Value=0  OutDataTypeStr=boolean
      settings: AttributesFormatString=DT: %<OutDataTypeStr>
  Out1 : Outport
  wires:
  Bus Selector6/1 -> Out1/1
  Bus Creator1/1 -> Bus Selector6/1
  x6/1 -> Bus Creator1/5  "wake"
  Bus Selector4/1 -> Bus Creator1/1  "<kl15>"
  In1/1 -> Bus Selector4/1
  In2/1 -> Bus Selector5/1
  Bus Selector5/1 -> Bus Creator1/2  "<RDY_H>"
  Bus Selector5/2 -> Bus Creator1/3  "<RDY_L>"
  x2/1 -> Bus Creator1/4  "stL2AscEn"

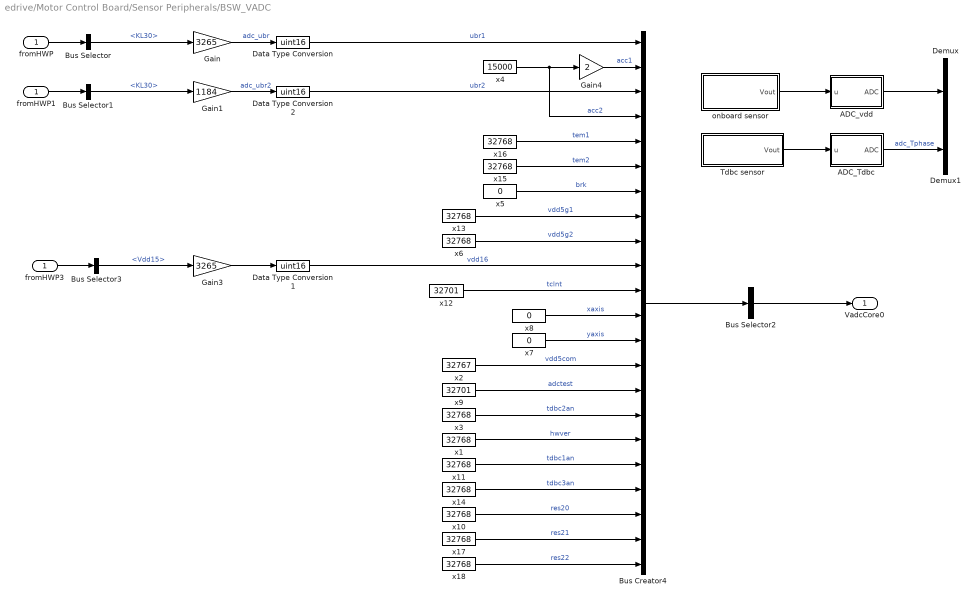
== system edrive/Motor Control Board/Sensor Peripherals/BSW_VADC ==
  fromHWP : Inport
  ADC_Tdbc : Subsystem
  ADC_vdd : Subsystem
  Bus Creator4 : BusCreator  Inputs=22
  Bus Selector : BusSelector  OutputSignals=KL30
  Bus Selector1 : BusSelector  OutputSignals=KL30
  Bus Selector2 : BusSelector  OutputSignals=ubr1,ubr2,vdd5g1,vdd5com,adctest,hwver,acc1,acc2,xaxis,yaxis,brk,tclnt,res20,res21,res22,tdbc1an,tdbc2an,tdbc3an,tem1,tem2,vdd16,vdd5g2  OutputAsBus=on
  Bus Selector3 : BusSelector  OutputSignals=Vdd15
  Data Type Conversion : DataTypeConversion  OutDataTypeStr=uint16  RndMeth=Convergent
  Data Type Conversion1 : DataTypeConversion  OutDataTypeStr=uint16  RndMeth=Convergent
  Data Type Conversion2 : DataTypeConversion  OutDataTypeStr=uint16  RndMeth=Convergent
  Demux : Demux
  Demux1 : Demux  Outputs=3
  Gain : Gain  Gain=3265
  Gain1 : Gain  Gain=1184
  Gain3 : Gain  Gain=3265
  Gain4 : Gain  Gain=2  OutDataTypeStr=uint16
  Tdbc sensor : Subsystem
  fromHWP1 : InportShadow
  fromHWP3 : InportShadow
  onboard sensor : Subsystem
  x{1,3,6,10..11,13..18} (11 alike) : Constant  Value=32768  OutDataTypeStr=uint16
      settings: AttributesFormatString=DT: %<OutDataTypeStr>
  x12 : Constant  Value=32701  OutDataTypeStr=uint16
      settings: AttributesFormatString=DT: %<OutDataTypeStr>
  x2 : Constant  Value=32767  OutDataTypeStr=uint16
      settings: AttributesFormatString=DT: %<OutDataTypeStr>
  x4 : Constant  Value=15000  OutDataTypeStr=uint16
      settings: AttributesFormatString=DT: %<OutDataTypeStr>
  x5 : Constant  Value=0  OutDataTypeStr=uint16
      settings: AttributesFormatString=DT: %<OutDataTypeStr>
  x7 : Constant  Value=0  OutDataTypeStr=uint16
      settings: AttributesFormatString=DT: %<OutDataTypeStr>
  x8 : Constant  Value=0  OutDataTypeStr=uint16
      settings: AttributesFormatString=DT: %<OutDataTypeStr>
  x9 : Constant  Value=32701  OutDataTypeStr=uint16
      settings: AttributesFormatString=DT: %<OutDataTypeStr>
  VadcCore0 : Outport
  wires:
  onboard sensor/1(Vout) -> ADC_vdd/1(u)
  Tdbc sensor/1(Vout) -> ADC_Tdbc/1(u)
  ADC_vdd/1(ADC) -> Demux/1
  ADC_Tdbc/1(ADC) -> Demux1/1  "adc_Tphase"
  Gain/1 -> Data Type Conversion/1  "adc_ubr"
  x16/1 -> Bus Creator4/5  "tem1"
  Gain1/1 -> Data Type Conversion2/1  "adc_ubr2"
  fromHWP/1 -> Bus Selector/1
  fromHWP1/1 -> Bus Selector1/1
  Bus Selector1/1 -> Gain1/1  "<KL30>"
  fromHWP3/1 -> Bus Selector3/1
  Bus Selector3/1 -> Gain3/1  "<Vdd15>"
  Gain3/1 -> Data Type Conversion1/1
  Bus Selector/1 -> Gain/1  "<KL30>"
  Data Type Conversion/1 -> Bus Creator4/1  "ubr1"
  Data Type Conversion2/1 -> Bus Creator4/3  "ubr2"
  x4/1 -> Bus Creator4/4, Gain4/1  "acc2"
  Gain4/1 -> Bus Creator4/2  "acc1"
  x15/1 -> Bus Creator4/6  "tem2"
  x5/1 -> Bus Creator4/7  "brk"
  x13/1 -> Bus Creator4/8  "vdd5g1"
  x6/1 -> Bus Creator4/9  "vdd5g2"
  Data Type Conversion1/1 -> Bus Creator4/10  "vdd16"
  x12/1 -> Bus Creator4/11  "tclnt"
  x8/1 -> Bus Creator4/12  "xaxis"
  x7/1 -> Bus Creator4/13  "yaxis"
  x2/1 -> Bus Creator4/14  "vdd5com"
  x9/1 -> Bus Creator4/15  "adctest"
  x3/1 -> Bus Creator4/16  "tdbc2an"
  x14/1 -> Bus Creator4/19  "tdbc3an"
  x11/1 -> Bus Creator4/18  "tdbc1an"
  x1/1 -> Bus Creator4/17  "hwver"
  Bus Creator4/1 -> Bus Selector2/1
  Bus Selector2/1 -> VadcCore0/1
  x18/1 -> Bus Creator4/22  "res22"
  x17/1 -> Bus Creator4/21  "res21"
  x10/1 -> Bus Creator4/20  "res20"

== system edrive/Motor Control Board/Sensor Peripherals/CDDResolver ==
  note: take the model data instead of the real cdd based on the real resolver output waveform
  note: Simplified resolver CDD in DSADC
  RslvrOut : Inport
  eleAngle : Inport  Port=2
  Rotor speed wm (rad/s) : Inport  Port=3
  Constant : Constant  Value=19000  OutDataTypeStr=int16
  Constant3 : Constant  Value=0  OutDataTypeStr=int16
  DTC{1..4} (4 alike) : DataTypeConversion  OutDataTypeStr=int16
  Delay1 : Delay  DelayLength=50  InitialCondition=0
  Gain : Gain  Gain=32768/pi
      settings: AttributesFormatString=|
      | -------------------
      | [0 2pi) to [0 65536)
  Gain1 : Gain  Gain=pmsm.RslvrPolePairs
      settings: AttributesFormatString=|
      | -------------------
      | resolver pole pairs
  Mux : Mux
  Mux1 : Mux  Inputs=2
  Terminator : Terminator
  "cos " : Fcn  Expr=cos(u)*29000
  sin : Fcn  Expr=sin(u)*29000
  Rslvr : Outport
  theta : Outport  Port=2
  wele : Outport  Port=3
  RslvrLv2 : Outport  Port=4
  wires:
  eleAngle/1 -> Delay1/1, Gain/1
  Gain1/1 -> DTC1/1
  Gain/1 -> DTC2/1
  DTC2/1 -> theta/1  "theta"
  DTC1/1 -> wele/1  "elew"
  Rotor speed wm (rad/s)/1 -> Gain1/1
  Mux/1 -> Rslvr/1  "dsadc_resolver"
  "cos "/1 -> Mux1/1, DTC3/1
  sin/1 -> Mux1/2, DTC4/1
  DTC3/1 -> Mux/1  "sin"
  DTC4/1 -> Mux/2  "cos"
  Constant/1 -> Mux/3  "Ext"
  Constant3/1 -> Mux/4  "ExtOffs"
  Delay1/1 -> "cos "/1, sin/1
  RslvrOut/1 -> Terminator/1
  Mux1/1 -> RslvrLv2/1

== system edrive/Motor Control Board/Sensor Peripherals/CDDResolverLv2 ==
  note: take the model data instead of the real cdd based on the real resolver output waveform
  note: Simplified resolver CDD in DSADC
  RslvrLv2 : Inport
  Constant : Constant  Value=32767  OutDataTypeStr=int16
  Constant1 : Constant  Value=32767  OutDataTypeStr=int16
  DTC{1..4} (4 alike) : DataTypeConversion  OutDataTypeStr=uint16
  Demux2 : Demux  Outputs=2
  Sum : Sum  Inputs=|++
  Sum1 : Sum  Inputs=|++
  SinH : Outport
  SinL : Outport  Port=2
  CosH : Outport  Port=3
  CosL : Outport  Port=4
  wires:
  Sum/1 -> DTC3/1
  DTC3/1 -> SinH/1  "SinH"
  Constant/1 -> Sum/2, DTC2/1
  RslvrLv2/1 -> Demux2/1
  Demux2/1 -> Sum/1
  DTC2/1 -> SinL/1  "SinL"
  Demux2/2 -> Sum1/1
  Constant1/1 -> Sum1/2, DTC4/1
  Sum1/1 -> DTC1/1
  DTC1/1 -> CosH/1  "CosH"
  DTC4/1 -> CosL/1  "CosL"

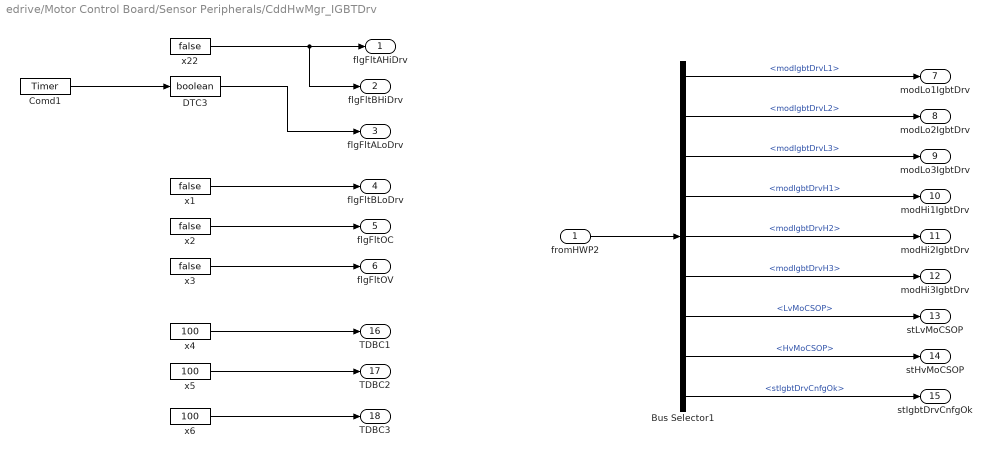
== system edrive/Motor Control Board/Sensor Peripherals/CddHwMgr_IGBTDrv ==
  fromHWP2 : Inport
  Bus Selector1 : BusSelector  OutputSignals=modIgbtDrvL1,modIgbtDrvL2,modIgbtDrvL3,modIgbtDrvH1,modIgbtDrvH2,modIgbtDrvH3,LvMoCSOP,HvMoCSOP,stIgbtDrvCnfgOk
  Comd1 : powerlib_extras/Control  Blocks/Timer  t="[ 0  0.3]"  e="[0  0]"
  DTC3 : DataTypeConversion  OutDataTypeStr=boolean
  x{1..3,22} (4 alike) : Constant  Value=false  OutDataTypeStr=boolean
      settings: AttributesFormatString=DT: %<OutDataTypeStr>
  x4 : Constant  Value=100  OutDataTypeStr=uint16
      settings: AttributesFormatString=DT: %<OutDataTypeStr>
  x5 : Constant  Value=100  OutDataTypeStr=uint16
      settings: AttributesFormatString=DT: %<OutDataTypeStr>
  x6 : Constant  Value=100  OutDataTypeStr=uint16
      settings: AttributesFormatString=DT: %<OutDataTypeStr>
  flgFltAHiDrv : Outport
  flgFltBHiDrv : Outport  Port=2
  flgFltALoDrv : Outport  Port=3
  flgFltBLoDrv : Outport  Port=4
  flgFltOC : Outport  Port=5
  flgFltOV : Outport  Port=6
  modLo1IgbtDrv : Outport  Port=7
  modLo2IgbtDrv : Outport  Port=8
  modLo3IgbtDrv : Outport  Port=9
  modHi1IgbtDrv : Outport  Port=10
  modHi2IgbtDrv : Outport  Port=11
  modHi3IgbtDrv : Outport  Port=12
  stLvMoCSOP : Outport  Port=13
  stHvMoCSOP : Outport  Port=14
  stIgbtDrvCnfgOk : Outport  Port=15
  TDBC1 : Outport  Port=16
  TDBC2 : Outport  Port=17
  TDBC3 : Outport  Port=18
  wires:
  x22/1 -> flgFltBHiDrv/1, flgFltAHiDrv/1
  x1/1 -> flgFltBLoDrv/1
  x2/1 -> flgFltOC/1
  Comd1/1 -> DTC3/1
  DTC3/1 -> flgFltALoDrv/1
  x3/1 -> flgFltOV/1
  fromHWP2/1 -> Bus Selector1/1
  Bus Selector1/1 -> modLo1IgbtDrv/1  "<modIgbtDrvL1>"
  Bus Selector1/2 -> modLo2IgbtDrv/1  "<modIgbtDrvL2>"
  Bus Selector1/3 -> modLo3IgbtDrv/1  "<modIgbtDrvL3>"
  Bus Selector1/4 -> modHi1IgbtDrv/1  "<modIgbtDrvH1>"
  Bus Selector1/5 -> modHi2IgbtDrv/1  "<modIgbtDrvH2>"
  Bus Selector1/6 -> modHi3IgbtDrv/1  "<modIgbtDrvH3>"
  Bus Selector1/7 -> stLvMoCSOP/1  "<LvMoCSOP>"
  Bus Selector1/8 -> stHvMoCSOP/1  "<HvMoCSOP>"
  Bus Selector1/9 -> stIgbtDrvCnfgOk/1  "<stIgbtDrvCnfgOk>"
  x5/1 -> TDBC2/1
  x4/1 -> TDBC1/1
  x6/1 -> TDBC3/1

== system edrive/Motor Control Board/Sensor Peripherals/Resolver ==
  angRaw : Inport
  excitatiion : Inport  Port=2
  Add : Sum  Inputs=+++
  BLWN2 : simulink/Sources/Band-Limited White Noise  Cov=[(0.005*pi)^2/10000000]  Ts=ctrlConst.TsSim  seed=[23341]
  Bus Creator : BusCreator  Inputs=2
  Constant1 : Constant  Value=-pi/2+0*pi  SampleTime=-1
  Constant2 : Constant  Value=2*pi  SampleTime=-1
  Gain1 : Gain  Gain=pmsm.RslvrPolePairs
      settings: AttributesFormatString=|
      | -------------------
      | resolver pole pairs:
      | %<Gain>
  Gain2 : Gain  Gain=pmsm.RslvrRatio
      settings: AttributesFormatString=|
      | -------------------
      | resolver pole pairs:
      | %<Gain>
  Math Function : Math  Operator=mod  SaturateOnIntegerOverflow=on
  Product : Product
  Product1 : Product
  Trigonometric Function : Trigonometry
  Trigonometric Function1 : Trigonometry  Operator=cos
  RslvrOut : Outport
  eleAngle : Outport  Port=2
  wires:
  Constant2/1 -> Math Function/2
  Math Function/1 -> Trigonometric Function1/1, eleAngle/1, Trigonometric Function/1
  Gain1/1 -> Add/1
  Add/1 -> Math Function/1
  Constant1/1 -> Add/2
  angRaw/1 -> Gain1/1
  BLWN2/1 -> Add/3
  Trigonometric Function/1 -> Product/1
  Trigonometric Function1/1 -> Product1/1
  Product/1 -> Bus Creator/1  "sinxsint"
  Product1/1 -> Bus Creator/2  "cosxsint"
  Bus Creator/1 -> Gain2/1
  Gain2/1 -> RslvrOut/1
  excitatiion/1 -> Product/2, Product1/2

== system edrive/Motor Control Board/Sensor Peripherals/current sensor ==
  note: Current Sensor
  Isense : Inport
  ADC Amps To Volts : Constant  Value=sensors.Current.AmpsToVolts
  ADC Bias Volts : Constant  Value=sensors.Current.BiasVolts
  Add Bias : Sum
  Product Amps To Volts : Product  RndMeth=Zero
  Vout : Outport
  wires:
  Add Bias/1 -> Vout/1
  Isense/1 -> Product Amps To Volts/1
  ADC Amps To Volts/1 -> Product Amps To Volts/2
  Product Amps To Volts/1 -> Add Bias/1
  ADC Bias Volts/1 -> Add Bias/2

== system edrive/Motor Control Board/Sensor Peripherals/udclink sensor ==
  note: UdcLink Sensor
  uSense : Inport
  facUdc2Volts : Gain  Gain=sensors.Dclink.VoltToVolt
  Vout : Outport
  wires:
  uSense/1 -> facUdc2Volts/1
  facUdc2Volts/1 -> Vout/1

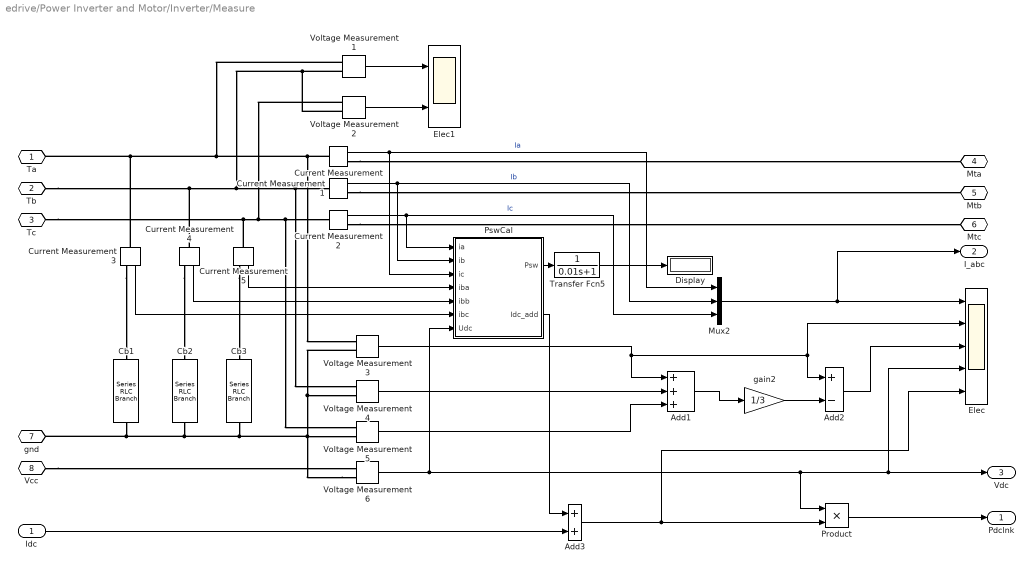
== system edrive/Power Inverter and Motor/Inverter/Measure ==
  Idc : Inport
  Add1 : Sum  Inputs=+++
  Add2 : Sum  Inputs=+-
  Add3 : Sum
  Cb1 : powerlib/Elements/Series RLC Branch  LConnTagsString=__new0  RConnTagsString=__new0  BranchType=RC  Resistance=100  Inductance=7e-9  SetiL0=off  InitialCurrent=0  Capacitance=10e-9  Setx0=on  InitialVoltage=0  Measurements=None
  Cb2 : powerlib/Elements/Series RLC Branch  LConnTagsString=__new0  RConnTagsString=__new0  BranchType=RC  Resistance=100  Inductance=7e-9  SetiL0=off  InitialCurrent=0  Capacitance=10e-9  Setx0=on  InitialVoltage=0  Measurements=None
  Cb3 : powerlib/Elements/Series RLC Branch  LConnTagsString=__new0  RConnTagsString=__new0  BranchType=RC  Resistance=100  Inductance=7e-9  SetiL0=off  InitialCurrent=0  Capacitance=10e-9  Setx0=on  InitialVoltage=0  Measurements=None
  Current Measurement{,1..5} (6 alike) : powerlib/Measurements/Current Measurement  Tag=PoWeRsYsTeMmEaSuReMeNt  PhasorSimulation=off  OutputType=Magnitude  PSBequivalent=0
  Display : Display
  Elec : Scope  NumInputPorts=5
  Elec1 : Scope  NumInputPorts=2
  Mux2 : Mux  Inputs=3
  Product : Product
  PswCal : MATLAB Function  TreatAsAtomicUnit=on
  Transfer Fcn5 : TransferFcn  Denominator=[0.01 1]
  Voltage Measurement{1..6} (6 alike) : powerlib/Measurements/Voltage Measurement  PhasorSimulation=off  OutputType=Complex  PSBequivalent=0
  gain2 : Gain  Gain=1/3  SaturateOnIntegerOverflow=on  OutDataTypeStr=Inherit: Same as input  ParamDataTypeStr=Inherit: Same as input
  Ta : PMIOPort  Port=1  Side=Left
  Tb : PMIOPort  Port=2  Side=Left
  Tc : PMIOPort  Port=3  Side=Left
  Mta : PMIOPort  Port=4  Side=Right
  Mtb : PMIOPort  Port=5  Side=Right
  Mtc : PMIOPort  Port=6  Side=Right
  gnd : PMIOPort  Port=7  Side=Left
  Vcc : PMIOPort  Port=8  Side=Left
  Pdclnk : Outport
  I_abc : Outport  Port=2
  Vdc : Outport  Port=3
  wires:
  Voltage Measurement3/1 -> Add1/1, Elec/2, Add2/1
  Voltage Measurement4/1 -> Add1/2
  Add1/1 -> gain2/1
  gain2/1 -> Add2/2
  Add2/1 -> Elec/3
  Idc/1 -> Add3/2
  Voltage Measurement5/1 -> Add1/3
  Voltage Measurement6/1 -> Product/1, Elec/4, Vdc/1, PswCal/7(Udc)
  Add3/1 -> Product/2, Elec/5
  Product/1 -> Pdclnk/1
  Current Measurement/1 -> Mux2/1, PswCal/3(ic)  "Ia"
  Current Measurement1/1 -> Mux2/2, PswCal/2(ib)  "Ib"
  Current Measurement2/1 -> Mux2/3, PswCal/1(ia)  "Ic"
  Mux2/1 -> I_abc/1, Elec/1
  Current Measurement5/1 -> PswCal/4(iba)
  Current Measurement4/1 -> PswCal/5(ibb)
  Current Measurement3/1 -> PswCal/6(ibc)
  PswCal/2(Idc_add) -> Add3/1
  Transfer Fcn5/1 -> Display/1
  PswCal/1(Psw) -> Transfer Fcn5/1
  Voltage Measurement1/1 -> Elec1/1
  Voltage Measurement2/1 -> Elec1/2
  connections:
  Tc/RConn1 -- Current Measurement5/LConn1 -- Voltage Measurement2/LConn1 -- Current Measurement2/LConn1 -- Voltage Measurement5/LConn1
  Tb/RConn1 -- Current Measurement4/LConn1 -- Voltage Measurement2/LConn2 -- Voltage Measurement1/LConn2 -- Current Measurement1/LConn1 -- Voltage Measurement4/LConn1
  Current Measurement/LConn1 -- Voltage Measurement1/LConn1 -- Current Measurement3/LConn1 -- Ta/RConn1 -- Voltage Measurement3/LConn1
  Current Measurement2/RConn1 -- Mtc/RConn1
  Current Measurement/RConn1 -- Mta/RConn1
  Current Measurement1/RConn1 -- Mtb/RConn1
  Voltage Measurement6/LConn2 -- Voltage Measurement3/LConn2 -- Voltage Measurement4/LConn2 -- Voltage Measurement5/LConn2 -- Cb2/RConn1 -- Cb1/RConn1 -- gnd/RConn1 -- Cb3/RConn1
  Vcc/RConn1 -- Voltage Measurement6/LConn1
  Current Measurement3/RConn1 -- Cb1/LConn1
  Current Measurement5/RConn1 -- Cb3/LConn1
  Current Measurement4/RConn1 -- Cb2/LConn1

== system edrive/Power Inverter and Motor/Motor_feishi150/PMSM ==
  In : Inport
  MotorMode : Inport  Port=2
  Continuous : Subsystem
  Continuous w input : Subsystem
  Measurement : Subsystem
  Powersystem : Subsystem
  Terminator3 : Terminator
  A : PMIOPort  Port=1  Side=Left
  B : PMIOPort  Port=2  Side=Left
  C : PMIOPort  Port=3  Side=Left
  m : Outport
  wires:
  [UabUbc] -> Continuous/1(v)
  In/1 -> Continuous w input/1(In)
  Measurement/1(Out1) -> m/1
  Continuous w input/3(the) -> Continuous/3(the)
  Continuous w input/1(m) -> Measurement/2(m_m)
  Continuous/3(Te) -> Continuous w input/2(Te)
  Continuous/2(m) -> Measurement/1(m_e)
  Continuous w input/2(we) -> Continuous/2(we)
  Continuous/1(i) -> Terminator3/1
  MotorMode/1 -> Continuous w input/3(MotorMode)
  connections:
  A/RConn1 -- Powersystem/LConn1
  B/RConn1 -- Powersystem/LConn2
  C/RConn1 -- Powersystem/LConn3

== system edrive/System Analysis/Measure/Subsystem ==
  iq : Inport
  id : Inport  Port=2
  Complex to Magnitude-Angle : ComplexToMagnitudeAngle
  Mux5 : Mux  Inputs=3
  Real-Imag to Complex : RealImagToComplex
  Terminator : Terminator
  Terminator2 : Terminator
  Transfer Fcn3 : TransferFcn  Denominator=[0.01 1]
  Cur. : Outport
  wires:
  Mux5/1 -> Cur./1
  id/1 -> Real-Imag to Complex/1, Mux5/1
  iq/1 -> Real-Imag to Complex/2, Mux5/2
  Real-Imag to Complex/1 -> Complex to Magnitude-Angle/1
  Complex to Magnitude-Angle/1 -> Mux5/3, Transfer Fcn3/1
  Complex to Magnitude-Angle/2 -> Terminator/1
  Transfer Fcn3/1 -> Terminator2/1

== system edrive/System Analysis/Measure/Subsystem1 ==
  vq : Inport
  vd : Inport  Port=2
  Complex to Magnitude-Angle : ComplexToMagnitudeAngle
  Mux5 : Mux
  Real-Imag to Complex : RealImagToComplex
  Terminator : Terminator
  Transfer Fcn3 : TransferFcn  Denominator=[0.01 1]
  Vol. : Outport
  wires:
  Mux5/1 -> Vol./1
  vd/1 -> Real-Imag to Complex/1, Mux5/1
  vq/1 -> Real-Imag to Complex/2, Mux5/2
  Real-Imag to Complex/1 -> Complex to Magnitude-Angle/1
  Complex to Magnitude-Angle/1 -> Transfer Fcn3/1, Mux5/3
  Complex to Magnitude-Angle/2 -> Terminator/1
  Transfer Fcn3/1 -> Mux5/4

== system edrive/System Analysis/Measure/Subsystem3 ==
  vd : Inport
  vq : Inport  Port=2
  id : Inport  Port=3
  iq : Inport  Port=4
  Add : Sum
  Constant : Constant  Value=3
  Product : Product
  Product2 : Product  RndMeth=Zero
  Product3 : Product  RndMeth=Zero
  Transfer Fcn5 : TransferFcn  Denominator=[0.01 1]
  E_Power : Outport
  wires:
  iq/1 -> Product3/2
  Product/1 -> Transfer Fcn5/1
  Product2/1 -> Add/1
  Constant/1 -> Product/2
  Product3/1 -> Add/2
  vq/1 -> Product3/1
  id/1 -> Product2/1
  Add/1 -> Product/1
  vd/1 -> Product2/2
  Transfer Fcn5/1 -> E_Power/1

== system edrive/System Analysis/Measure/Subsystem4 ==
  In1 : Inport
  In2 : Inport  Port=2
  Data Type Conversion : DataTypeConversion  OutDataTypeStr=double
  Gain4 : Gain  Gain=30/pi  SaturateOnIntegerOverflow=on  OutDataTypeStr=Inherit: Same as input  ParamDataTypeStr=Inherit: Same as input
  Subsystem2 : Subsystem
  Torque : Outport
  speed : Outport  Port=2
  M_Power : Outport  Port=3
  wires:
  In1/1 -> Gain4/1, Subsystem2/2(wm)
  Subsystem2/1(Power1) -> M_Power/1
  Gain4/1 -> speed/1
  In2/1 -> Subsystem2/1(Te), Data Type Conversion/1
  Data Type Conversion/1 -> Torque/1

== system edrive/Motor Control Board/GTM/SVPWMtoDuty/Generate pulse pattern ==
  TuHi_On : Inport
  TuHi_Off : Inport  Port=2
  GTM_Hi : MATLAB Function
  Triangle : simulink/Sources/Repeating Sequence  rep_seq_t=[0 1/Fc]  rep_seq_y=[0 1/Fc]
  TuHi : Outport
  wires:
  Triangle/1 -> GTM_Hi/1(Cnt)
  TuHi_On/1 -> GTM_Hi/2(tiOn)
  TuHi_Off/1 -> GTM_Hi/3(tiOff)
  GTM_Hi/1(Port) -> TuHi/1
